simulink library "sm_trackV_lib_belt_underc_elem"  (R2026a)
settings: Solver=VariableStepAuto
undefined symbols (not defined in the file): Excv, P00, P01, P02, P03, P04, P05, P06, P07, P08, P09, P10, P11, P12, P13, P14, P15, P16, P17, P18, P19, P20, Trac, X, Y, Z
libraries: sm_lib x193, $bdroot x42
(part 1 of 5)
Description:
  | Copyright 2024-2026 The MathWorks, Inc.
settings Model: Creator=smiller  LastModifiedBy=smiller

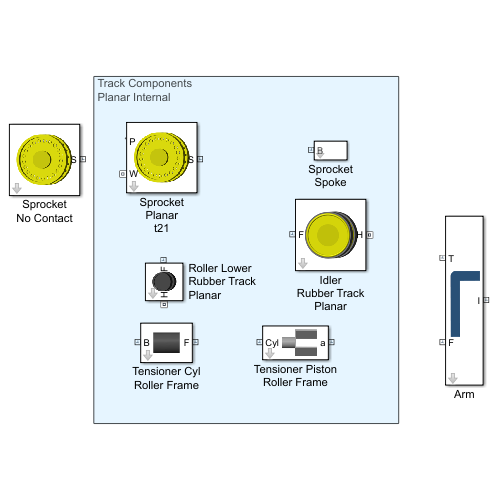
[thumbnail: Simulink's stored preview of the top-level diagram]
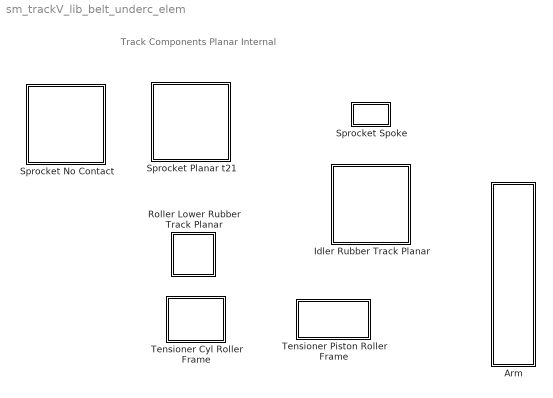
== system sm_trackV_lib_belt_underc_elem ==
  note: Track Components
      | Planar Internal
  Arm : Subsystem  mask(Idler Arm, Tracked Vehicle){arm_idlerc=Trac.IdlerArm.Pivot_to_Idler, arm_tens_x=Trac.IdlerArm.Pivot_to_TensionerX, arm_tens_y=Trac.IdlerArm.Pivot_to_TensionerY, arm_wid=Trac.IdlerArm.wid, arm_thk=Trac.IdlerArm.thk, arm_rho=Trac.IdlerArm.rho, arm_clr=Trac.IdlerArm.clr, arm_opc=Trac.IdlerArm.opc}
      mask prompts: arm_idlerc "Offset Pivot to Idler Center (m)"; arm_tens_x "Offset Pivot to Tensioner Long.  (m)"; arm_tens_y "Offset Pivot to Tensioner Vert.  (m)"; arm_wid "Idler Arm Width (m)"; arm_thk "Idler Arm Thickness (m)"; arm_rho "Idler Arm Density (kg/m^3)"; arm_clr "Idler Arm Color [R G B] (0-1)"; arm_opc "Idler Arm Opacity (0-1)"
      mask help: Models hinged idler arm for tracked vehicle. Connects idler wheel rotation axis to pivot point on lower frame and tensioner bracket.
      mask init:
      | upDown = 180*(ge(arm_tens_y,0));
      mask DialogControl Container4 Prompt: Idler Arm
      mask Display: image('sm_idler_arm_IMAGE.png')
  Idler Rubber Track Planar : Subsystem  mask(Idler, Belt Track, Planar Contact){idler_rad=Trac.IdlerF.rad, idler_len=Trac.IdlerF.len, wheel_clr=Trac.IdlerF.Wheel.clr, rim_rad=Trac.IdlerF.Rim.rad, rim_hub_rad=Trac.IdlerF.Rim.hub_rad, rim_xc=Trac.IdlerF.Rim.rim_xc, idler_rho=Trac.IdlerF.rho, idler_opc=Trac.IdlerF.opc, idler_clr=Trac.IdlerF.clr, idler_axle_rad=Trac.IdlerF.Axle.rad, idler_axle_len=Trac.IdlerF.Axle.len, idler_axle_rho=Trac.IdlerF.Axle.rho, idler_axle_opc=Trac.IdlerF.Axle.opc, idler_axle_clr=Trac.IdlerF.Axle.clr, idler_contgeo_clr=Trac.IdlerF.belt_contact.clr, idler_contgeo_opc=Trac.IdlerF.belt_contact.opc}
      mask prompts: idler_rad "Radius (m)"; idler_len "Length (m)"; wheel_clr "Wheel Color [R G B] (0-1)"; rim_rad "Radius (m)"; rim_hub_rad "Hub Radius (m)"; rim_xc "Cross Section [x y] (m)"; idler_rho "Density (kg/m^3)"; idler_opc "Opacity (0-1)"; idler_clr "Color [R G B] (0-1)"; idler_axle_rad "Radius (m)"; idler_axle_len "Length (m)"; idler_axle_rho "Density (kg/m^3)"; idler_axle_opc "Opacity (0-1)"; idler_axle_clr "Color [R G B] (0-1)"; idler_contgeo_clr "Color [R G B] (0-1)"; idler_contgeo_opc "Opacity (0-1)"
      mask help: Models idler on a rubber belt. Includes gap so lugs on belt can pass between rollers. Contact geometry assumes contact with belt is planar.
      mask init:
      | wheel_xc = [...
      |             rim_rad     -idler_len/2;
      |             idler_rad   -idler_len/2;
      |             idler_rad   idler_len/2;
      |             rim_rad     idler_len/2;
      |             ];
      mask DialogControl cont_idler_roller Prompt: Roller
      mask DialogControl cont_roller_rim Prompt: Rim
      mask DialogControl cont_idler_axle Prompt: Axle
      mask DialogControl cont_contact_geo_lower Prompt: Contact Geometry
      mask Display: image('sm_belt_idler_IMAGE.png');
  Roller Lower Rubber Track Planar : Subsystem  mask(Lower Roller, Belt Track, Planar Contact){roller_lower_rad=Trac.Roller.Lower.rad, roller_lower_len=Trac.Roller.Lower.len, roller_lower_rho=Trac.Roller.Lower.rho, roller_lower_clr=Trac.Roller.Lower.clr, roller_lower_opc=Trac.Roller.Lower.opc, roller_lower_rim_thk=Trac.Roller.Lower.rim_thk, roller_lower_rim_len=Trac.Roller.Lower.rim_len, roller_lower_axle_rad=Trac.Roller.Lower.Axle.rad, roller_lower_axle_len=Trac.Roller.Lower.Axle.len, roller_lower_axle_rho=Trac.Roller.Lower.Axle.rho, roller_lower_axle_opc=Trac.Roller.Lower.Axle.opc, roller_lower_axle_clr=Trac.Roller.Lower.Axle.clr, roller_lower_contgeo_clr=Trac.Roller.Lower.belt_contact.clr, roller_lower_contgeo_opc=Trac.Roller.Lower.belt_contact.opc}
      mask prompts: roller_lower_rad "Radius (m)"; roller_lower_len "Length (m)"; roller_lower_rho "Density (kg/m^3)"; roller_lower_clr "Color [R G B] (0-1)"; roller_lower_opc "Opacity (0-1)"; roller_lower_rim_thk "Thickness (m)"; roller_lower_rim_len "Length (m)"; roller_lower_axle_rad "Radius (m)"; roller_lower_axle_len "Length (m)"; roller_lower_axle_rho "Density (kg/m^3)"; roller_lower_axle_opc "Opacity (0-1)"; roller_lower_axle_clr "Color [R G B] (0-1)"; roller_lower_contgeo_clr "Color [R G B] (0-1)"; roller_lower_contgeo_opc "Opacity (0-1)"
      mask help: Models roller for use on rubber belt. Includes gap so lugs on belt can pass through. Contact geometry assumes contact with belt is planar.
      mask init:
      | roller_xc = [...
      |     0 -roller_lower_len/2+roller_lower_rim_len;...
      |     roller_lower_rad-roller_lower_rim_thk -roller_lower_len/2+roller_lower_rim_len;...
      |     roller_lower_rad-roller_lower_rim_thk -roller_lower_len/2;...
      |     roller_lower_rad                      -roller_lower_len/2;...
      |     roller_lower_rad                       roller_lower_len/2;...
      |     roller_lower_rad-roller_lower_rim_thk  roller_lower_len/2;...
      |     0                                      roller_lower_len/2];
      mask DialogControl cont_roller_lower Prompt: Roller
      mask DialogControl cont_rollerL_rim Prompt: Rim
      mask DialogControl cont_roller_lower_axle Prompt: Axle
      mask DialogControl cont_contact_geo_lower Prompt: Contact Geometry
      mask Display: image('sm_belt_roller_IMAGE.png');
  Sprocket No Contact : Subsystem  mask(Sprocket Wheel, Belt Track, Planar Contact){sprk_wid_roll=Trac.Sprocket.Roller.wid, sprk_rad_roll=Trac.Sprocket.Roller.rad, sprk_opc=Trac.Sprocket.Roller.opc, sprk_clr=Trac.Sprocket.Roller.clr, sprk_rad_pitch=Trac.Sprocket.Spoke.pitch_rad, sprk_spoke_rad=Trac.Sprocket.Spoke.rad, sprk_spoke_len=Trac.Sprocket.Spoke.len, sprk_spoke_num=Trac.Sprocket.nSpokes, sprk_spoke_clr=Trac.Sprocket.Spoke.clr, sprk_spoke_opc=Trac.Sprocket.Spoke.opc, rim_spoke_xc=Trac.Sprocket.Rim.spoke_xc, rim_thk=Trac.Sprocket.Rim.thk, rim_ir=Trac.Sprocket.Rim.rad_inner}
      mask prompts: sprk_wid_roll "Roller Width (m)"; sprk_rad_roll "Rolling Radius (m)"; sprk_opc "Roller Opacity (0-1)"; sprk_clr "Roller Color [R G B] (0-1)"; sprk_rad_pitch "Pitch Radius (m)"; sprk_spoke_rad "Radius (m)"; sprk_spoke_len "Length (m)"; sprk_spoke_num "Number of Spokes"; sprk_spoke_clr "Spoke Color [R G B] (0-1)"; sprk_spoke_opc "Spoke Opacity (0-1)"; rim_spoke_xc "Spoke Cross Section [x y] (m)"; rim_thk "Thickness (m)"; rim_ir "Inner Radius (m)"
      mask help: Models sprocket for belt track. Pins contact lugs on belt, rollers contact belt. Contact geometry assumes contact with belt and lugs is planar.
      mask DialogControl cont_sprkt Prompt: Sprocket
      mask DialogControl cont_sprk_roller Prompt: Roller
      mask DialogControl cont_sprk_spoke Prompt: Spoke
      mask DialogControl cont_sprk_rim Prompt: Rim
      mask Display: image('sm_belt_sprocket_IMAGE.png')
  Sprocket Planar t21 : Subsystem  mask(Sprocket Wheel, Belt Track, Planar Contact){sprk_wid_roll=Trac.Sprocket.Roller.wid, sprk_rad_roll=Trac.Sprocket.Roller.rad, sprk_opc=Trac.Sprocket.Roller.opc, sprk_clr=Trac.Sprocket.Roller.clr, sprk_rad_pitch=Trac.Sprocket.Spoke.pitch_rad, sprk_spoke_rad=Trac.Sprocket.Spoke.rad, sprk_spoke_len=Trac.Sprocket.Spoke.len, sprk_spoke_num=Trac.Sprocket.nSpokes, sprk_spoke_clr=Trac.Sprocket.Spoke.clr, sprk_spoke_opc=Trac.Sprocket.Spoke.opc, rim_spoke_xc=Trac.Sprocket.Rim.spoke_xc, rim_thk=Trac.Sprocket.Rim.thk, rim_ir=Trac.Sprocket.Rim.rad_inner, sprk_contgeo_roller_clr=Trac.Sprocket.roller_contact.clr, sprk_contgeo_roller_opc=Trac.Sprocket.roller_contact.opc, sprk_contgeo_spoke_clr=Trac.Sprocket.spoke_contact.clr, sprk_contgeo_spoke_opc=Trac.Sprocket.spoke_contact.opc}
      mask prompts: sprk_wid_roll "Roller Width (m)"; sprk_rad_roll "Rolling Radius (m)"; sprk_opc "Roller Opacity (0-1)"; sprk_clr "Roller Color [R G B] (0-1)"; sprk_rad_pitch "Pitch Radius (m)"; sprk_spoke_rad "Radius (m)"; sprk_spoke_len "Length (m)"; sprk_spoke_num "Number of Spokes"; sprk_spoke_clr "Spoke Color [R G B] (0-1)"; sprk_spoke_opc "Spoke Opacity (0-1)"; rim_spoke_xc "Spoke Cross Section [x y] (m)"; rim_thk "Thickness (m)"; rim_ir "Inner Radius (m)"; sprk_contgeo_roller_clr "Roller Color [R G B] (0-1)"; sprk_contgeo_roller_opc "Roller Opacity (0-1)"; sprk_contgeo_spoke_clr "Spoke Color [R G B] (0-1)"; sprk_contgeo_spoke_opc "Spoke Opacity (0-1)"
      mask help: Models sprocket for belt track. Pins contact lugs on belt, rollers contact belt. Contact geometry assumes contact with belt and lugs is planar.
      mask DialogControl cont_sprkt Prompt: Sprocket
      mask DialogControl cont_sprk_roller Prompt: Roller
      mask DialogControl cont_sprk_spoke Prompt: Spoke
      mask DialogControl cont_sprk_rim Prompt: Rim
      mask DialogControl cont_sprk_contgeo Prompt: Contact Geometry
      mask Display: image('sm_belt_sprocket_IMAGE.png')
  Sprocket Spoke : Subsystem  mask(Spoke on Sprocket Wheel){spoke_xc=Trac.Sprocket.xc_spoke, spoke_thk=Trac.Sprocket.spoke_thk, spoke_clr=Trac.Sprocket.Roller.clr, spoke_opc=Trac.Sprocket.Roller.opc, sprk_pin_len=Trac.Sprocket.Spoke.len}
      mask prompts: spoke_xc "Spoke Cross-Section [x y] (m)"; spoke_thk "Spoke Thickness (m)"; spoke_clr "Spoke Color [R G B] (0-1)"; spoke_opc "Spoke Color (0-1)"; sprk_pin_len "Sprocket Pin Length (m)"
      mask help: Models geometry of spoke in sprocket wheel. Spoke has pin at midpoint outer edge.
      mask init:
      | spoke_offset = (sprk_pin_len+spoke_thk)/2;
      mask TypeOptions spoke_xc: Spoke nz/ExtrusionCrossSection | Spoke pz/ExtrusionCrossSection
      mask TypeOptions spoke_thk: Spoke nz/ExtrusionLength | Spoke pz/ExtrusionLength
      mask TypeOptions spoke_clr: Spoke nz/GraphicDiffuseColor | Spoke pz/GraphicDiffuseColor
      mask TypeOptions spoke_opc: Spoke nz/GraphicOpacity | Spoke pz/GraphicOpacity
  Tensioner Cyl Roller Frame : Subsystem  mask(Tensioner Cylinder){cyl_rad=Excv.Idler.Tensioner.cyl.rad, cyl_len=Excv.Idler.Tensioner.cyl.len, cyl_rho=Excv.Idler.Tensioner.cyl.rho, cyl_clr=Excv.Idler.Tensioner.cyl.clr, cyl_opc=Excv.Idler.Tensioner.cyl.opc}
      mask prompts: cyl_rad "Radius (m)"; cyl_len "Length (m)"; cyl_rho "Density (kg/m^3)"; cyl_clr "Color [R G B] (0-1)"; cyl_opc "Opacity (0-1)"
      mask help: Models tensioner cylinder in undercarriage.
      mask DialogControl cont_cyl Prompt: Cylinder
      mask Display: image('sm_chain_tensioner_cyl_IMAGE.png');
  Tensioner Piston Roller Frame : Subsystem  mask(Tensioner Piston and Bracket){pist_rad=Excv.Idler.Tensioner.piston.rad, pist_len=Excv.Idler.Tensioner.piston.len, pist_rho=Excv.Idler.Tensioner.piston.rho, pist_clr=Excv.Idler.Tensioner.piston.clr, pist_opc=Excv.Idler.Tensioner.piston.opc, br_height=Excv.Idler.Tensioner.bracket.height, br_length=Excv.Idler.Tensioner.bracket.len, br_width=Excv.Idler.Tensioner.bracket.wid, br_rho=Excv.Idler.Tensioner.bracket.rho, br_thk=Excv.Idler.Tensioner.bracket.thk, br_clr=Excv.Idler.Tensioner.bracket.clr, br_opc=Excv.Idler.Tensioner.bracket.opc}
      mask prompts: pist_rad "Radius (m)"; pist_len "Length (m)"; pist_rho "Density (kg/m^3)"; pist_clr "Color [R G B] (0-1)"; pist_opc "Opacity (0.1)"; br_height "Height (m)"; br_length "Length (m)"; br_width "Width (m)"; br_rho "Density (kg/m^3)"; br_thk "Thickness (m)"; br_clr "Color [R G B] (0-1)"; br_opc "Opacity (0.1)"
      mask help: Models tensioner piston and bracket in undercarriage.
      mask DialogControl cont_piston Prompt: Piston
      mask DialogControl cont_bracket Prompt: Bracket
      mask Display: image('sm_chain_tensioner_piston_IMAGE.png');

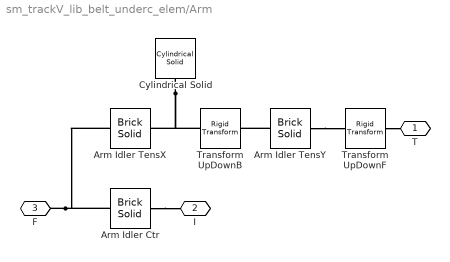
== system sm_trackV_lib_belt_underc_elem/Arm ==
  Arm Idler Ctr : sm_lib/Body Elements/Brick Solid  BrickDimensions=[arm_idlerc arm_wid arm_thk]  BrickDimensionsUnits=m  ExportEntireGeometry=off  InertiaType=CalculateFromGeometry  BasedOnType=Density  Density=arm_rho  DensityUnits=kg/m^3  Mass=1  MassUnits=kg  CenterOfMass=[0 0 0]  CenterOfMassUnits=m  MomentsOfInertia=[1 1 1]  MomentsOfInertiaUnits=kg*m^2  ProductsOfInertia=[0 0 0]  ProductsOfInertiaUnits=kg*m^2  GraphicType=FromGeometry  MarkerShape=Sphere  MarkerSize=10  GraphicVisPropType=SimpleVisualProperties  GraphicDiffuseColor=arm_clr  GraphicOpacity=arm_opc  GraphicSpecularColor=[0.5 0.5 0.5 1.0]  GraphicAmbientColor=[0.15 0.15 0.15 1.0]  GraphicEmissiveColor=[0.0 0.0 0.0 1.0]  GraphicShininess=75  DoExposeReferenceFrame=off  SerializedFrames=<Frames><Frame><Id>Frame1</Id><Value><Name>B</Name><Origin><Source>GeometricFeature</Source><FeatureName>-x surface</FeatureName></Origin><PrimaryAxis><DefinedDirection>+Z</DefinedDirection><Source>ReferenceFrame</Source><SourceDirection>+Z</SourceDirection><FeatureName></FeatureName></PrimaryAxis><SecondaryAxis><DefinedDirection>+X</DefinedDirection><Source>ReferenceFrame</Source><SourceDirection>+X</SourceDirection><FeatureName></FeatureName></SecondaryAxis></Value></Frame><Frame><Id>Frame2</Id><Value><Name>F</Name><Origin><Source>GeometricFeature</Source><FeatureName>+x surface</FeatureName></Origin><PrimaryAxis><DefinedDirection>+Z</DefinedDirection><Source>ReferenceFrame</Source><SourceDirection>+Z</SourceDirection><FeatureName></FeatureName></PrimaryAxis><SecondaryAxis><DefinedDirection>+X</DefinedDirection><Source>ReferenceFrame</Source><SourceDirection>+X</SourceDirection><FeatureName></FeatureName></SecondaryAxis></Value></Frame></Frames>
  Arm Idler TensX : sm_lib/Body Elements/Brick Solid  BrickDimensions=[arm_tens_x arm_wid arm_thk]  BrickDimensionsUnits=m  ExportEntireGeometry=off  InertiaType=CalculateFromGeometry  BasedOnType=Density  Density=arm_rho  DensityUnits=kg/m^3  Mass=1  MassUnits=kg  CenterOfMass=[0 0 0]  CenterOfMassUnits=m  MomentsOfInertia=[1 1 1]  MomentsOfInertiaUnits=kg*m^2  ProductsOfInertia=[0 0 0]  ProductsOfInertiaUnits=kg*m^2  GraphicType=FromGeometry  MarkerShape=Sphere  MarkerSize=10  GraphicVisPropType=SimpleVisualProperties  GraphicDiffuseColor=arm_clr  GraphicOpacity=arm_opc  GraphicSpecularColor=[0.5 0.5 0.5 1.0]  GraphicAmbientColor=[0.15 0.15 0.15 1.0]  GraphicEmissiveColor=[0.0 0.0 0.0 1.0]  GraphicShininess=75  DoExposeReferenceFrame=off  SerializedFrames=<Frames><Frame><Id>Frame1</Id><Value><Name>B</Name><Origin><Source>GeometricFeature</Source><FeatureName>-x surface</FeatureName></Origin><PrimaryAxis><DefinedDirection>+Z</DefinedDirection><Source>ReferenceFrame</Source><SourceDirection>+Z</SourceDirection><FeatureName></FeatureName></PrimaryAxis><SecondaryAxis><DefinedDirection>+X</DefinedDirection><Source>ReferenceFrame</Source><SourceDirection>+X</SourceDirection><FeatureName></FeatureName></SecondaryAxis></Value></Frame><Frame><Id>Frame2</Id><Value><Name>F</Name><Origin><Source>GeometricFeature</Source><FeatureName>+x surface</FeatureName></Origin><PrimaryAxis><DefinedDirection>+Z</DefinedDirection><Source>ReferenceFrame</Source><SourceDirection>+Z</SourceDirection><FeatureName></FeatureName></PrimaryAxis><SecondaryAxis><DefinedDirection>+X</DefinedDirection><Source>ReferenceFrame</Source><SourceDirection>+X</SourceDirection><FeatureName></FeatureName></SecondaryAxis></Value></Frame></Frames>
  Arm Idler TensY : sm_lib/Body Elements/Brick Solid  BrickDimensions=[arm_wid abs(arm_tens_y) arm_thk]  BrickDimensionsUnits=m  ExportEntireGeometry=off  InertiaType=CalculateFromGeometry  BasedOnType=Density  Density=arm_rho  DensityUnits=kg/m^3  Mass=1  MassUnits=kg  CenterOfMass=[0 0 0]  CenterOfMassUnits=m  MomentsOfInertia=[1 1 1]  MomentsOfInertiaUnits=kg*m^2  ProductsOfInertia=[0 0 0]  ProductsOfInertiaUnits=kg*m^2  GraphicType=FromGeometry  MarkerShape=Sphere  MarkerSize=10  GraphicVisPropType=SimpleVisualProperties  GraphicDiffuseColor=arm_clr  GraphicOpacity=arm_opc  GraphicSpecularColor=[0.5 0.5 0.5 1.0]  GraphicAmbientColor=[0.15 0.15 0.15 1.0]  GraphicEmissiveColor=[0.0 0.0 0.0 1.0]  GraphicShininess=75  DoExposeReferenceFrame=off  SerializedFrames=<Frames><Frame><Id>Frame1</Id><Value><Name>B</Name><Origin><Source>GeometricFeature</Source><FeatureName>+y surface</FeatureName></Origin><PrimaryAxis><DefinedDirection>+Z</DefinedDirection><Source>ReferenceFrame</Source><SourceDirection>+Z</SourceDirection><FeatureName></FeatureName></PrimaryAxis><SecondaryAxis><DefinedDirection>+X</DefinedDirection><Source>ReferenceFrame</Source><SourceDirection>+X</SourceDirection><FeatureName></FeatureName></SecondaryAxis></Value></Frame><Frame><Id>Frame2</Id><Value><Name>F</Name><Origin><Source>GeometricFeature</Source><FeatureName>-y surface</FeatureName></Origin><PrimaryAxis><DefinedDirection>+Z</DefinedDirection><Source>ReferenceFrame</Source><SourceDirection>+Z</SourceDirection><FeatureName></FeatureName></PrimaryAxis><SecondaryAxis><DefinedDirection>+X</DefinedDirection><Source>ReferenceFrame</Source><SourceDirection>+X</SourceDirection><FeatureName></FeatureName></SecondaryAxis></Value></Frame></Frames>
  Cylindrical Solid : sm_lib/Body Elements/Cylindrical Solid  CylinderRadius=arm_wid/2  CylinderRadiusUnits=m  CylinderLength=arm_thk  CylinderLengthUnits=m  ExportEntireGeometry=off  InertiaType=CalculateFromGeometry  BasedOnType=Density  Density=arm_rho  DensityUnits=kg/m^3  Mass=1  MassUnits=kg  CenterOfMass=[0 0 0]  CenterOfMassUnits=m  MomentsOfInertia=[1 1 1]  MomentsOfInertiaUnits=kg*m^2  ProductsOfInertia=[0 0 0]  ProductsOfInertiaUnits=kg*m^2  GraphicType=FromGeometry  MarkerShape=Sphere  MarkerSize=10  GraphicVisPropType=SimpleVisualProperties  GraphicDiffuseColor=arm_clr  GraphicOpacity=arm_opc  GraphicSpecularColor=[0.5 0.5 0.5 1.0]  GraphicAmbientColor=[0.15 0.15 0.15 1.0]  GraphicEmissiveColor=[0.0 0.0 0.0 1.0]  GraphicShininess=75  DoExposeReferenceFrame=on  SerializedFrames=<Frames/>
  Transform UpDownB : sm_lib/Frames and Transforms/Rigid Transform  RotationMethod=StandardAxis  FollAlignAxisA=+X  BaseAlignAxisA=+Y  FollAlignAxisB=+Y  BaseAlignAxisB=+Z  RotationStandardAxis=+X  RotationAngle=upDown  RotationAngleUnits=deg  RotationArbitraryAxis=[0 0 1]  RotationSequenceAxes=FollowerAxes  RotationSequence=XYX  RotationSequenceAngles=[0 0 0]  RotationSequenceAnglesUnits=deg  RotationMatrix=[1 0 0; 0 1 0; 0 0 1]  Quaternion=[1 0 0 0]  TranslationMethod=None  TranslationCartesianOffset=[0 0 0]  TranslationCartesianOffsetUnits=m  TranslationStandardAxis=+Z  TranslationStandardOffset=0  TranslationStandardOffsetUnits=m  TranslationROffset=0  TranslationROffsetUnits=m  TranslationThetaOffset=0  TranslationThetaOffsetUnits=deg  TranslationZOffset=0  TranslationZOffsetUnits=m
  Transform UpDownF : sm_lib/Frames and Transforms/Rigid Transform  RotationMethod=StandardAxis  FollAlignAxisA=+X  BaseAlignAxisA=+Y  FollAlignAxisB=+Y  BaseAlignAxisB=+Z  RotationStandardAxis=+X  RotationAngle=upDown  RotationAngleUnits=deg  RotationArbitraryAxis=[0 0 1]  RotationSequenceAxes=FollowerAxes  RotationSequence=XYX  RotationSequenceAngles=[0 0 0]  RotationSequenceAnglesUnits=deg  RotationMatrix=[1 0 0; 0 1 0; 0 0 1]  Quaternion=[1 0 0 0]  TranslationMethod=None  TranslationCartesianOffset=[0 0 0]  TranslationCartesianOffsetUnits=m  TranslationStandardAxis=+Z  TranslationStandardOffset=0  TranslationStandardOffsetUnits=m  TranslationROffset=0  TranslationROffsetUnits=m  TranslationThetaOffset=0  TranslationThetaOffsetUnits=deg  TranslationZOffset=0  TranslationZOffsetUnits=m
  T : PMIOPort  Side=Left
  I : PMIOPort  Port=2  Side=Right
  F : PMIOPort  Port=3  Side=Left
  connections:
  Cylindrical Solid/RConn1 -- Arm Idler TensX/RConn1 -- Transform UpDownB/LConn1
  Arm Idler Ctr/RConn1 -- I/RConn1
  F/RConn1 -- Arm Idler TensX/LConn1 -- Arm Idler Ctr/LConn1
  Arm Idler TensY/RConn1 -- Transform UpDownF/RConn1
  Transform UpDownF/LConn1 -- T/RConn1
  Arm Idler TensY/LConn1 -- Transform UpDownB/RConn1

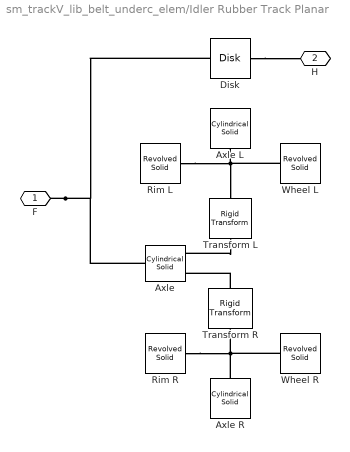
== system sm_trackV_lib_belt_underc_elem/Idler Rubber Track Planar ==
  Axle : sm_lib/Body Elements/Cylindrical Solid  CylinderRadius=idler_axle_rad  CylinderRadiusUnits=m  CylinderLength=idler_axle_len  CylinderLengthUnits=m  ExportEntireGeometry=off  InertiaType=CalculateFromGeometry  BasedOnType=Density  Density=idler_axle_rho  DensityUnits=kg/m^3  Mass=1  MassUnits=kg  CenterOfMass=[0 0 0]  CenterOfMassUnits=m  MomentsOfInertia=[1 1 1]  MomentsOfInertiaUnits=kg*m^2  ProductsOfInertia=[0 0 0]  ProductsOfInertiaUnits=kg*m^2  GraphicType=FromGeometry  MarkerShape=Sphere  MarkerSize=10  GraphicVisPropType=SimpleVisualProperties  GraphicDiffuseColor=idler_axle_clr  GraphicOpacity=idler_axle_opc  GraphicSpecularColor=[0.5 0.5 0.5 1.0]  GraphicAmbientColor=[0.15 0.15 0.15 1.0]  GraphicEmissiveColor=[0.0 0.0 0.0 1.0]  GraphicShininess=75  DoExposeReferenceFrame=on  SerializedFrames=<Frames><Frame><Id>Frame1</Id><Value><Name>F</Name><Origin><Source>GeometricFeature</Source><FeatureName>top surface</FeatureName></Origin><PrimaryAxis><DefinedDirection>+Z</DefinedDirection><Source>ReferenceFrame</Source><SourceDirection>+Z</SourceDirection><FeatureName></FeatureName></PrimaryAxis><SecondaryAxis><DefinedDirection>+X</DefinedDirection><Source>ReferenceFrame</Source><SourceDirection>+X</SourceDirection><FeatureName></FeatureName></SecondaryAxis></Value></Frame><Frame><Id>Frame2</Id><Value><Name>B</Name><Origin><Source>GeometricFeature</Source><FeatureName>bottom surface</FeatureName></Origin><PrimaryAxis><DefinedDirection>+Z</DefinedDirection><Source>ReferenceFrame</Source><SourceDirection>+Z</SourceDirection><FeatureName></FeatureName></PrimaryAxis><SecondaryAxis><DefinedDirection>+X</DefinedDirection><Source>ReferenceFrame</Source><SourceDirection>+X</SourceDirection><FeatureName></FeatureName></SecondaryAxis></Value></Frame></Frames>
  Axle L : sm_lib/Body Elements/Cylindrical Solid  CylinderRadius=rim_hub_rad  CylinderRadiusUnits=m  CylinderLength=max(rim_xc(:,2))*2  CylinderLengthUnits=m  ExportEntireGeometry=off  InertiaType=CalculateFromGeometry  BasedOnType=Density  Density=idler_rho  DensityUnits=kg/m^3  Mass=1  MassUnits=kg  CenterOfMass=[0 0 0]  CenterOfMassUnits=m  MomentsOfInertia=[1 1 1]  MomentsOfInertiaUnits=kg*m^2  ProductsOfInertia=[0 0 0]  ProductsOfInertiaUnits=kg*m^2  GraphicType=FromGeometry  MarkerShape=Sphere  MarkerSize=10  GraphicVisPropType=SimpleVisualProperties  GraphicDiffuseColor=idler_clr*0.9  GraphicOpacity=idler_opc  GraphicSpecularColor=[0.5 0.5 0.5 1.0]  GraphicAmbientColor=[0.15 0.15 0.15 1.0]  GraphicEmissiveColor=[0.0 0.0 0.0 1.0]  GraphicShininess=75  DoExposeReferenceFrame=on  SerializedFrames=<Frames/>
  Axle R : sm_lib/Body Elements/Cylindrical Solid  CylinderRadius=rim_hub_rad  CylinderRadiusUnits=m  CylinderLength=max(rim_xc(:,2))*2  CylinderLengthUnits=m  ExportEntireGeometry=off  InertiaType=CalculateFromGeometry  BasedOnType=Density  Density=idler_rho  DensityUnits=kg/m^3  Mass=1  MassUnits=kg  CenterOfMass=[0 0 0]  CenterOfMassUnits=m  MomentsOfInertia=[1 1 1]  MomentsOfInertiaUnits=kg*m^2  ProductsOfInertia=[0 0 0]  ProductsOfInertiaUnits=kg*m^2  GraphicType=FromGeometry  MarkerShape=Sphere  MarkerSize=10  GraphicVisPropType=SimpleVisualProperties  GraphicDiffuseColor=idler_clr*0.9  GraphicOpacity=idler_opc  GraphicSpecularColor=[0.5 0.5 0.5 1.0]  GraphicAmbientColor=[0.15 0.15 0.15 1.0]  GraphicEmissiveColor=[0.0 0.0 0.0 1.0]  GraphicShininess=75  DoExposeReferenceFrame=on  SerializedFrames=<Frames/>
  Disk : sm_lib/Curves and Surfaces/Disk  Radius=idler_rad  RadiusUnits=m  GraphicType=FromGeometry  GraphicVisPropType=SimpleVisualProperties  GraphicDiffuseColor=idler_contgeo_clr  GraphicOpacity=idler_contgeo_opc  GraphicSpecularColor=[0.5 0.5 0.5 1.0]  GraphicAmbientColor=[0.15 0.15 0.15 1.0]  GraphicEmissiveColor=[0.0 0.0 0.0 1.0]  GraphicShininess=75
  Rim L : sm_lib/Body Elements/Revolved Solid  RevolutionCrossSection=rim_xc  RevolutionCrossSectionUnits=m  RevolutionExtent=Full  RevolutionAngle=180  RevolutionAngleUnits=deg  ExportConvexHullGeometry=off  InertiaType=CalculateFromGeometry  BasedOnType=Density  Density=idler_rho  DensityUnits=kg/m^3  Mass=1  MassUnits=kg  CenterOfMass=[0 0 0]  CenterOfMassUnits=m  MomentsOfInertia=[1 1 1]  MomentsOfInertiaUnits=kg*m^2  ProductsOfInertia=[0 0 0]  ProductsOfInertiaUnits=kg*m^2  GraphicType=FromGeometry  MarkerShape=Sphere  MarkerSize=10  GraphicVisPropType=SimpleVisualProperties  GraphicDiffuseColor=idler_clr  GraphicOpacity=idler_opc  GraphicSpecularColor=[0.5 0.5 0.5 1.0]  GraphicAmbientColor=[0.15 0.15 0.15 1.0]  GraphicEmissiveColor=[0.0 0.0 0.0 1.0]  GraphicShininess=75  DoExposeReferenceFrame=on  SerializedFrames=<Frames/>
  Rim R : sm_lib/Body Elements/Revolved Solid  RevolutionCrossSection=rim_xc  RevolutionCrossSectionUnits=m  RevolutionExtent=Full  RevolutionAngle=180  RevolutionAngleUnits=deg  ExportConvexHullGeometry=off  InertiaType=CalculateFromGeometry  BasedOnType=Density  Density=idler_rho  DensityUnits=kg/m^3  Mass=1  MassUnits=kg  CenterOfMass=[0 0 0]  CenterOfMassUnits=m  MomentsOfInertia=[1 1 1]  MomentsOfInertiaUnits=kg*m^2  ProductsOfInertia=[0 0 0]  ProductsOfInertiaUnits=kg*m^2  GraphicType=FromGeometry  MarkerShape=Sphere  MarkerSize=10  GraphicVisPropType=SimpleVisualProperties  GraphicDiffuseColor=idler_clr  GraphicOpacity=idler_opc  GraphicSpecularColor=[0.5 0.5 0.5 1.0]  GraphicAmbientColor=[0.15 0.15 0.15 1.0]  GraphicEmissiveColor=[0.0 0.0 0.0 1.0]  GraphicShininess=75  DoExposeReferenceFrame=on  SerializedFrames=<Frames/>
  Transform L : sm_lib/Frames and Transforms/Rigid Transform  RotationMethod=None  FollAlignAxisA=+X  BaseAlignAxisA=+Y  FollAlignAxisB=+Y  BaseAlignAxisB=+Z  RotationStandardAxis=+Z  RotationAngle=0.0  RotationAngleUnits=deg  RotationArbitraryAxis=[0 0 1]  RotationSequenceAxes=FollowerAxes  RotationSequence=XYX  RotationSequenceAngles=[0 0 0]  RotationSequenceAnglesUnits=deg  RotationMatrix=[1 0 0; 0 1 0; 0 0 1]  Quaternion=[1 0 0 0]  TranslationMethod=StandardAxis  TranslationCartesianOffset=[0 0 0]  TranslationCartesianOffsetUnits=m  TranslationStandardAxis=+Z  TranslationStandardOffset=idler_len/2  TranslationStandardOffsetUnits=m  TranslationROffset=0  TranslationROffsetUnits=m  TranslationThetaOffset=0  TranslationThetaOffsetUnits=deg  TranslationZOffset=0  TranslationZOffsetUnits=m
  Transform R : sm_lib/Frames and Transforms/Rigid Transform  RotationMethod=None  FollAlignAxisA=+X  BaseAlignAxisA=+Y  FollAlignAxisB=+Y  BaseAlignAxisB=+Z  RotationStandardAxis=+Z  RotationAngle=0.0  RotationAngleUnits=deg  RotationArbitraryAxis=[0 0 1]  RotationSequenceAxes=FollowerAxes  RotationSequence=XYX  RotationSequenceAngles=[0 0 0]  RotationSequenceAnglesUnits=deg  RotationMatrix=[1 0 0; 0 1 0; 0 0 1]  Quaternion=[1 0 0 0]  TranslationMethod=StandardAxis  TranslationCartesianOffset=[0 0 0]  TranslationCartesianOffsetUnits=m  TranslationStandardAxis=-Z  TranslationStandardOffset=idler_len/2  TranslationStandardOffsetUnits=m  TranslationROffset=0  TranslationROffsetUnits=m  TranslationThetaOffset=0  TranslationThetaOffsetUnits=deg  TranslationZOffset=0  TranslationZOffsetUnits=m
  Wheel L : sm_lib/Body Elements/Revolved Solid  RevolutionCrossSection=wheel_xc  RevolutionCrossSectionUnits=m  RevolutionExtent=Full  RevolutionAngle=180  RevolutionAngleUnits=deg  ExportConvexHullGeometry=off  InertiaType=CalculateFromGeometry  BasedOnType=Density  Density=idler_rho  DensityUnits=kg/m^3  Mass=1  MassUnits=kg  CenterOfMass=[0 0 0]  CenterOfMassUnits=m  MomentsOfInertia=[1 1 1]  MomentsOfInertiaUnits=kg*m^2  ProductsOfInertia=[0 0 0]  ProductsOfInertiaUnits=kg*m^2  GraphicType=FromGeometry  MarkerShape=Sphere  MarkerSize=10  GraphicVisPropType=SimpleVisualProperties  GraphicDiffuseColor=wheel_clr  GraphicOpacity=idler_opc  GraphicSpecularColor=[0.5 0.5 0.5 1.0]  GraphicAmbientColor=[0.15 0.15 0.15 1.0]  GraphicEmissiveColor=[0.0 0.0 0.0 1.0]  GraphicShininess=75  DoExposeReferenceFrame=on  SerializedFrames=<Frames/>
  Wheel R : sm_lib/Body Elements/Revolved Solid  RevolutionCrossSection=wheel_xc  RevolutionCrossSectionUnits=m  RevolutionExtent=Full  RevolutionAngle=180  RevolutionAngleUnits=deg  ExportConvexHullGeometry=off  InertiaType=CalculateFromGeometry  BasedOnType=Density  Density=idler_rho  DensityUnits=kg/m^3  Mass=1  MassUnits=kg  CenterOfMass=[0 0 0]  CenterOfMassUnits=m  MomentsOfInertia=[1 1 1]  MomentsOfInertiaUnits=kg*m^2  ProductsOfInertia=[0 0 0]  ProductsOfInertiaUnits=kg*m^2  GraphicType=FromGeometry  MarkerShape=Sphere  MarkerSize=10  GraphicVisPropType=SimpleVisualProperties  GraphicDiffuseColor=wheel_clr  GraphicOpacity=idler_opc  GraphicSpecularColor=[0.5 0.5 0.5 1.0]  GraphicAmbientColor=[0.15 0.15 0.15 1.0]  GraphicEmissiveColor=[0.0 0.0 0.0 1.0]  GraphicShininess=75  DoExposeReferenceFrame=on  SerializedFrames=<Frames/>
  F : PMIOPort  Side=Left
  H : PMIOPort  Port=2  Side=Right
  connections:
  Transform L/LConn1 -- Axle/LConn1
  Transform R/LConn1 -- Axle/LConn2
  F/RConn1 -- Disk/LConn1 -- Axle/RConn1
  Disk/RConn1 -- H/RConn1
  Rim L/RConn1 -- Transform L/RConn1 -- Axle L/RConn1 -- Wheel L/RConn1
  Wheel R/RConn1 -- Axle R/RConn1 -- Transform R/RConn1 -- Rim R/RConn1

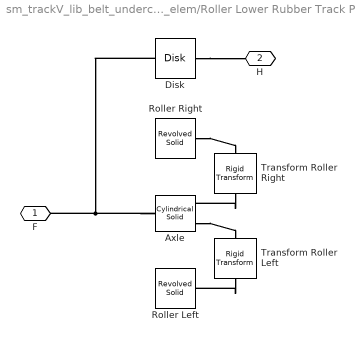
== system sm_trackV_lib_belt_underc_elem/Roller Lower Rubber Track Planar ==
  Axle : sm_lib/Body Elements/Cylindrical Solid  CylinderRadius=roller_lower_axle_rad  CylinderRadiusUnits=m  CylinderLength=roller_lower_axle_len  CylinderLengthUnits=m  ExportEntireGeometry=off  InertiaType=CalculateFromGeometry  BasedOnType=Density  Density=roller_lower_axle_rho  DensityUnits=kg/m^3  Mass=1  MassUnits=kg  CenterOfMass=[0 0 0]  CenterOfMassUnits=m  MomentsOfInertia=[1 1 1]  MomentsOfInertiaUnits=kg*m^2  ProductsOfInertia=[0 0 0]  ProductsOfInertiaUnits=kg*m^2  GraphicType=FromGeometry  MarkerShape=Sphere  MarkerSize=10  GraphicVisPropType=SimpleVisualProperties  GraphicDiffuseColor=roller_lower_axle_clr  GraphicOpacity=roller_lower_axle_opc  GraphicSpecularColor=[0.5 0.5 0.5 1.0]  GraphicAmbientColor=[0.15 0.15 0.15 1.0]  GraphicEmissiveColor=[0.0 0.0 0.0 1.0]  GraphicShininess=75  DoExposeReferenceFrame=on  SerializedFrames=<Frames><Frame><Id>Frame1</Id><Value><Name>F</Name><Origin><Source>GeometricFeature</Source><FeatureName>top surface</FeatureName></Origin><PrimaryAxis><DefinedDirection>+Z</DefinedDirection><Source>ReferenceFrame</Source><SourceDirection>+Z</SourceDirection><FeatureName></FeatureName></PrimaryAxis><SecondaryAxis><DefinedDirection>+X</DefinedDirection><Source>ReferenceFrame</Source><SourceDirection>+X</SourceDirection><FeatureName></FeatureName></SecondaryAxis></Value></Frame><Frame><Id>Frame2</Id><Value><Name>B</Name><Origin><Source>GeometricFeature</Source><FeatureName>bottom surface</FeatureName></Origin><PrimaryAxis><DefinedDirection>+Z</DefinedDirection><Source>ReferenceFrame</Source><SourceDirection>+Z</SourceDirection><FeatureName></FeatureName></PrimaryAxis><SecondaryAxis><DefinedDirection>+X</DefinedDirection><Source>ReferenceFrame</Source><SourceDirection>+X</SourceDirection><FeatureName></FeatureName></SecondaryAxis></Value></Frame></Frames>
  Disk : sm_lib/Curves and Surfaces/Disk  Radius=roller_lower_rad  RadiusUnits=m  GraphicType=FromGeometry  GraphicVisPropType=SimpleVisualProperties  GraphicDiffuseColor=roller_lower_contgeo_clr  GraphicOpacity=roller_lower_contgeo_opc  GraphicSpecularColor=[0.5 0.5 0.5 1.0]  GraphicAmbientColor=[0.15 0.15 0.15 1.0]  GraphicEmissiveColor=[0.0 0.0 0.0 1.0]  GraphicShininess=75
  Roller Left : sm_lib/Body Elements/Revolved Solid  RevolutionCrossSection=roller_xc  RevolutionCrossSectionUnits=m  RevolutionExtent=Full  RevolutionAngle=180  RevolutionAngleUnits=deg  ExportConvexHullGeometry=off  InertiaType=CalculateFromGeometry  BasedOnType=Density  Density=roller_lower_rho  DensityUnits=kg/m^3  Mass=1  MassUnits=kg  CenterOfMass=[0 0 0]  CenterOfMassUnits=m  MomentsOfInertia=[1 1 1]  MomentsOfInertiaUnits=kg*m^2  ProductsOfInertia=[0 0 0]  ProductsOfInertiaUnits=kg*m^2  GraphicType=FromGeometry  MarkerShape=Sphere  MarkerSize=10  GraphicVisPropType=SimpleVisualProperties  GraphicDiffuseColor=roller_lower_clr  GraphicOpacity=roller_lower_opc  GraphicSpecularColor=[0.5 0.5 0.5 1.0]  GraphicAmbientColor=[0.15 0.15 0.15 1.0]  GraphicEmissiveColor=[0.0 0.0 0.0 1.0]  GraphicShininess=75  DoExposeReferenceFrame=on  SerializedFrames=<Frames/>
  Roller Right : sm_lib/Body Elements/Revolved Solid  RevolutionCrossSection=roller_xc  RevolutionCrossSectionUnits=m  RevolutionExtent=Full  RevolutionAngle=180  RevolutionAngleUnits=deg  ExportConvexHullGeometry=off  InertiaType=CalculateFromGeometry  BasedOnType=Density  Density=roller_lower_rho  DensityUnits=kg/m^3  Mass=1  MassUnits=kg  CenterOfMass=[0 0 0]  CenterOfMassUnits=m  MomentsOfInertia=[1 1 1]  MomentsOfInertiaUnits=kg*m^2  ProductsOfInertia=[0 0 0]  ProductsOfInertiaUnits=kg*m^2  GraphicType=FromGeometry  MarkerShape=Sphere  MarkerSize=10  GraphicVisPropType=SimpleVisualProperties  GraphicDiffuseColor=roller_lower_clr  GraphicOpacity=roller_lower_opc  GraphicSpecularColor=[0.5 0.5 0.5 1.0]  GraphicAmbientColor=[0.15 0.15 0.15 1.0]  GraphicEmissiveColor=[0.0 0.0 0.0 1.0]  GraphicShininess=75  DoExposeReferenceFrame=on  SerializedFrames=<Frames/>
  Transform Roller Left : sm_lib/Frames and Transforms/Rigid Transform  RotationMethod=None  FollAlignAxisA=+X  BaseAlignAxisA=+Y  FollAlignAxisB=+Y  BaseAlignAxisB=+Z  RotationStandardAxis=+Z  RotationAngle=0.0  RotationAngleUnits=deg  RotationArbitraryAxis=[0 0 1]  RotationSequenceAxes=FollowerAxes  RotationSequence=XYX  RotationSequenceAngles=[0 0 0]  RotationSequenceAnglesUnits=deg  RotationMatrix=[1 0 0; 0 1 0; 0 0 1]  Quaternion=[1 0 0 0]  TranslationMethod=StandardAxis  TranslationCartesianOffset=[0 0 0]  TranslationCartesianOffsetUnits=m  TranslationStandardAxis=+Z  TranslationStandardOffset=roller_lower_len/2  TranslationStandardOffsetUnits=m  TranslationROffset=0  TranslationROffsetUnits=m  TranslationThetaOffset=0  TranslationThetaOffsetUnits=deg  TranslationZOffset=0  TranslationZOffsetUnits=m
  Transform Roller Right : sm_lib/Frames and Transforms/Rigid Transform  RotationMethod=StandardAxis  FollAlignAxisA=+X  BaseAlignAxisA=+Y  FollAlignAxisB=+Y  BaseAlignAxisB=+Z  RotationStandardAxis=+X  RotationAngle=180  RotationAngleUnits=deg  RotationArbitraryAxis=[0 0 1]  RotationSequenceAxes=FollowerAxes  RotationSequence=XYX  RotationSequenceAngles=[0 0 0]  RotationSequenceAnglesUnits=deg  RotationMatrix=[1 0 0; 0 1 0; 0 0 1]  Quaternion=[1 0 0 0]  TranslationMethod=StandardAxis  TranslationCartesianOffset=[0 0 0]  TranslationCartesianOffsetUnits=m  TranslationStandardAxis=+Z  TranslationStandardOffset=roller_lower_len/2  TranslationStandardOffsetUnits=m  TranslationROffset=0  TranslationROffsetUnits=m  TranslationThetaOffset=0  TranslationThetaOffsetUnits=deg  TranslationZOffset=0  TranslationZOffsetUnits=m
  F : PMIOPort  Side=Left
  H : PMIOPort  Port=2  Side=Right
  connections:
  Disk/RConn1 -- H/RConn1
  Axle/RConn1 -- Disk/LConn1 -- F/RConn1
  Axle/LConn2 -- Transform Roller Left/RConn1
  Transform Roller Right/LConn1 -- Axle/LConn1
  Roller Right/RConn1 -- Transform Roller Right/RConn1
  Transform Roller Left/LConn1 -- Roller Left/RConn1

== system sm_trackV_lib_belt_underc_elem/Sprocket No Contact ==
  Roller : Subsystem
  Spokes : Subsystem
  S : PMIOPort  Side=Right
  connections:
  Spokes/LConn21 -- Roller/RConn21
  Spokes/LConn20 -- Roller/RConn20
  Spokes/LConn19 -- Roller/RConn19
  Spokes/LConn18 -- Roller/RConn18
  Spokes/LConn17 -- Roller/RConn17
  Spokes/LConn16 -- Roller/RConn16
  Spokes/LConn15 -- Roller/RConn15
  Spokes/LConn14 -- Roller/RConn14
  Spokes/LConn13 -- Roller/RConn13
  Spokes/LConn12 -- Roller/RConn12
  Spokes/LConn11 -- Roller/RConn11
  Spokes/LConn10 -- Roller/RConn10
  Spokes/LConn9 -- Roller/RConn9
  Spokes/LConn8 -- Roller/RConn8
  Spokes/LConn7 -- Roller/RConn7
  Spokes/LConn6 -- Roller/RConn6
  Spokes/LConn5 -- Roller/RConn5
  Spokes/LConn4 -- Roller/RConn4
  Spokes/LConn3 -- Roller/RConn3
  Spokes/LConn2 -- Roller/RConn2
  Spokes/LConn1 -- Roller/RConn1
  Roller/LConn1 -- S/RConn1

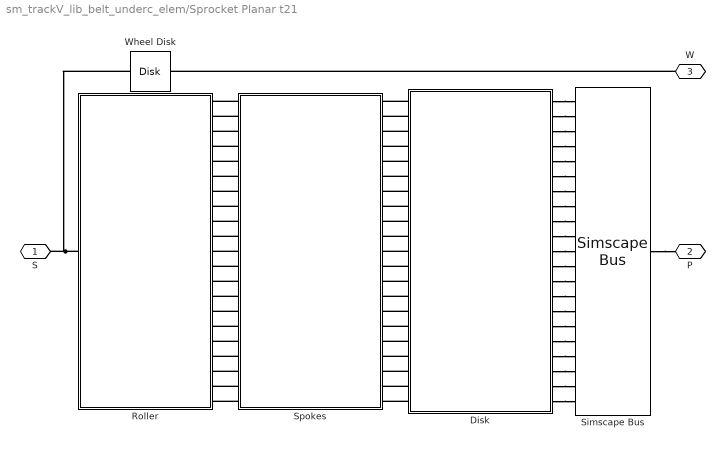
== system sm_trackV_lib_belt_underc_elem/Sprocket Planar t21 ==
  Disk : Subsystem
  Roller : Subsystem
  Simscape Bus : SimscapeBus  HierarchyStrings=P00;P01;P02;P03;P04;P05;P06;P07;P08;P09;P10;P11;P12;P13;P14;P15;P16;P17;P18;P19;P20
  Spokes : Subsystem
  Wheel Disk : sm_lib/Curves and Surfaces/Disk  Radius=sprk_rad_roll  RadiusUnits=m  GraphicType=FromGeometry  GraphicVisPropType=SimpleVisualProperties  GraphicDiffuseColor=sprk_contgeo_roller_clr  GraphicOpacity=sprk_contgeo_roller_opc  GraphicSpecularColor=[0.5 0.5 0.5 1.0]  GraphicAmbientColor=[0.15 0.15 0.15 1.0]  GraphicEmissiveColor=[0.0 0.0 0.0 1.0]  GraphicShininess=75
  S : PMIOPort  Side=Right
  P : PMIOPort  Port=2  Side=Left
  W : PMIOPort  Port=3  Side=Left
  connections:
  Simscape Bus/RConn1 -- P/RConn1
  W/RConn1 -- Wheel Disk/RConn1
  Wheel Disk/LConn1 -- Roller/LConn1 -- S/RConn1
  Spokes/LConn1 -- Roller/RConn1
  Spokes/LConn2 -- Roller/RConn2
  Spokes/LConn3 -- Roller/RConn3
  Spokes/LConn4 -- Roller/RConn4
  Spokes/LConn5 -- Roller/RConn5
  Spokes/LConn6 -- Roller/RConn6
  Spokes/LConn7 -- Roller/RConn7
  Spokes/LConn8 -- Roller/RConn8
  Spokes/LConn9 -- Roller/RConn9
  Spokes/LConn10 -- Roller/RConn10
  Spokes/LConn11 -- Roller/RConn11
  Spokes/LConn12 -- Roller/RConn12
  Spokes/LConn13 -- Roller/RConn13
  Spokes/LConn14 -- Roller/RConn14
  Spokes/LConn15 -- Roller/RConn15
  Spokes/LConn16 -- Roller/RConn16
  Spokes/LConn17 -- Roller/RConn17
  Spokes/LConn18 -- Roller/RConn18
  Spokes/LConn19 -- Roller/RConn19
  Spokes/LConn20 -- Roller/RConn20
  Spokes/LConn21 -- Roller/RConn21
  Disk/LConn1 -- Spokes/RConn1
  Disk/RConn1 -- Simscape Bus/LConn1
  Disk/LConn2 -- Spokes/RConn2
  Disk/RConn2 -- Simscape Bus/LConn2
  Disk/LConn3 -- Spokes/RConn3
  Disk/RConn3 -- Simscape Bus/LConn3
  Disk/LConn4 -- Spokes/RConn4
  Disk/RConn4 -- Simscape Bus/LConn4
  Disk/LConn5 -- Spokes/RConn5
  Disk/RConn5 -- Simscape Bus/LConn5
  Disk/LConn6 -- Spokes/RConn6
  Disk/RConn6 -- Simscape Bus/LConn6
  Disk/LConn7 -- Spokes/RConn7
  Disk/RConn7 -- Simscape Bus/LConn7
  Disk/LConn8 -- Spokes/RConn8
  Disk/RConn8 -- Simscape Bus/LConn8
  Disk/LConn9 -- Spokes/RConn9
  Disk/RConn9 -- Simscape Bus/LConn9
  Disk/LConn10 -- Spokes/RConn10
  Disk/RConn10 -- Simscape Bus/LConn10
  Disk/LConn11 -- Spokes/RConn11
  Disk/RConn11 -- Simscape Bus/LConn11
  Disk/LConn12 -- Spokes/RConn12
  Disk/RConn12 -- Simscape Bus/LConn12
  Disk/LConn13 -- Spokes/RConn13
  Disk/RConn13 -- Simscape Bus/LConn13
  Disk/LConn14 -- Spokes/RConn14
  Disk/RConn14 -- Simscape Bus/LConn14
  Disk/LConn15 -- Spokes/RConn15
  Disk/RConn15 -- Simscape Bus/LConn15
  Disk/LConn16 -- Spokes/RConn16
  Disk/RConn16 -- Simscape Bus/LConn16
  Disk/LConn17 -- Spokes/RConn17
  Disk/RConn17 -- Simscape Bus/LConn17
  Disk/LConn18 -- Spokes/RConn18
  Disk/RConn18 -- Simscape Bus/LConn18
  Disk/LConn19 -- Spokes/RConn19
  Disk/RConn19 -- Simscape Bus/LConn19
  Disk/LConn20 -- Spokes/RConn20
  Disk/RConn20 -- Simscape Bus/LConn20
  Disk/LConn21 -- Spokes/RConn21
  Disk/RConn21 -- Simscape Bus/LConn21

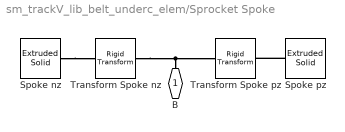
== system sm_trackV_lib_belt_underc_elem/Sprocket Spoke ==
  Spoke nz : sm_lib/Body Elements/Extruded Solid  ExtrusionType=General  PolygonNumSides=3  PolygonOuterRadius=1  PolygonOuterRadiusUnits=m  ExportEntireGeometry=off  ExtrusionCrossSection=spoke_xc  ExtrusionCrossSectionUnits=m  ExportConvexHullGeometry=off  ExtrusionLength=spoke_thk  ExtrusionLengthUnits=m  InertiaType=CalculateFromGeometry  BasedOnType=Density  Density=1000  DensityUnits=kg/m^3  Mass=1  MassUnits=kg  CenterOfMass=[0 0 0]  CenterOfMassUnits=m  MomentsOfInertia=[1 1 1]  MomentsOfInertiaUnits=kg*m^2  ProductsOfInertia=[0 0 0]  ProductsOfInertiaUnits=kg*m^2  GraphicType=FromGeometry  MarkerShape=Sphere  MarkerSize=10  GraphicVisPropType=SimpleVisualProperties  GraphicDiffuseColor=spoke_clr  GraphicOpacity=spoke_opc  GraphicSpecularColor=[0.5 0.5 0.5 1.0]  GraphicAmbientColor=[0.15 0.15 0.15 1.0]  GraphicEmissiveColor=[0.0 0.0 0.0 1.0]  GraphicShininess=75  DoExposeReferenceFrame=on  SerializedFrames=<Frames/>
  Spoke pz : sm_lib/Body Elements/Extruded Solid  ExtrusionType=General  PolygonNumSides=3  PolygonOuterRadius=1  PolygonOuterRadiusUnits=m  ExportEntireGeometry=off  ExtrusionCrossSection=spoke_xc  ExtrusionCrossSectionUnits=m  ExportConvexHullGeometry=off  ExtrusionLength=spoke_thk  ExtrusionLengthUnits=m  InertiaType=CalculateFromGeometry  BasedOnType=Density  Density=1000  DensityUnits=kg/m^3  Mass=1  MassUnits=kg  CenterOfMass=[0 0 0]  CenterOfMassUnits=m  MomentsOfInertia=[1 1 1]  MomentsOfInertiaUnits=kg*m^2  ProductsOfInertia=[0 0 0]  ProductsOfInertiaUnits=kg*m^2  GraphicType=FromGeometry  MarkerShape=Sphere  MarkerSize=10  GraphicVisPropType=SimpleVisualProperties  GraphicDiffuseColor=spoke_clr  GraphicOpacity=spoke_opc  GraphicSpecularColor=[0.5 0.5 0.5 1.0]  GraphicAmbientColor=[0.15 0.15 0.15 1.0]  GraphicEmissiveColor=[0.0 0.0 0.0 1.0]  GraphicShininess=75  DoExposeReferenceFrame=on  SerializedFrames=<Frames/>
  Transform Spoke nz : sm_lib/Frames and Transforms/Rigid Transform  RotationMethod=None  FollAlignAxisA=+X  BaseAlignAxisA=+Y  FollAlignAxisB=+Y  BaseAlignAxisB=+Z  RotationStandardAxis=+Z  RotationAngle=0.0  RotationAngleUnits=deg  RotationArbitraryAxis=[0 0 1]  RotationSequenceAxes=FollowerAxes  RotationSequence=XYX  RotationSequenceAngles=[0 0 0]  RotationSequenceAnglesUnits=deg  RotationMatrix=[1 0 0; 0 1 0; 0 0 1]  Quaternion=[1 0 0 0]  TranslationMethod=StandardAxis  TranslationCartesianOffset=[0 0 0]  TranslationCartesianOffsetUnits=m  TranslationStandardAxis=+Z  TranslationStandardOffset=-spoke_offset  TranslationStandardOffsetUnits=m  TranslationROffset=0  TranslationROffsetUnits=m  TranslationThetaOffset=0  TranslationThetaOffsetUnits=deg  TranslationZOffset=0  TranslationZOffsetUnits=m
  Transform Spoke pz : sm_lib/Frames and Transforms/Rigid Transform  RotationMethod=None  FollAlignAxisA=+X  BaseAlignAxisA=+Y  FollAlignAxisB=+Y  BaseAlignAxisB=+Z  RotationStandardAxis=+Z  RotationAngle=0.0  RotationAngleUnits=deg  RotationArbitraryAxis=[0 0 1]  RotationSequenceAxes=FollowerAxes  RotationSequence=XYX  RotationSequenceAngles=[0 0 0]  RotationSequenceAnglesUnits=deg  RotationMatrix=[1 0 0; 0 1 0; 0 0 1]  Quaternion=[1 0 0 0]  TranslationMethod=StandardAxis  TranslationCartesianOffset=[0 0 0]  TranslationCartesianOffsetUnits=m  TranslationStandardAxis=+Z  TranslationStandardOffset=spoke_offset  TranslationStandardOffsetUnits=m  TranslationROffset=0  TranslationROffsetUnits=m  TranslationThetaOffset=0  TranslationThetaOffsetUnits=deg  TranslationZOffset=0  TranslationZOffsetUnits=m
  B : PMIOPort  Side=Left
  connections:
  Spoke nz/RConn1 -- Transform Spoke nz/RConn1
  Transform Spoke nz/LConn1 -- Transform Spoke pz/LConn1 -- B/RConn1
  Spoke pz/RConn1 -- Transform Spoke pz/RConn1

== system sm_trackV_lib_belt_underc_elem/Tensioner Cyl Roller Frame ==
  Cylinder : sm_lib/Body Elements/Cylindrical Solid  CylinderRadius=cyl_rad  CylinderRadiusUnits=m  CylinderLength=cyl_len  CylinderLengthUnits=m  ExportEntireGeometry=off  InertiaType=CalculateFromGeometry  BasedOnType=Density  Density=cyl_rho  DensityUnits=kg/m^3  Mass=1  MassUnits=kg  CenterOfMass=[0 0 0]  CenterOfMassUnits=m  MomentsOfInertia=[1 1 1]  MomentsOfInertiaUnits=kg*m^2  ProductsOfInertia=[0 0 0]  ProductsOfInertiaUnits=kg*m^2  GraphicType=FromGeometry  MarkerShape=Sphere  MarkerSize=10  GraphicVisPropType=SimpleVisualProperties  GraphicDiffuseColor=cyl_clr  GraphicOpacity=cyl_opc  GraphicSpecularColor=[0.5 0.5 0.5 1.0]  GraphicAmbientColor=[0.15 0.15 0.15 1.0]  GraphicEmissiveColor=[0.0 0.0 0.0 1.0]  GraphicShininess=75  DoExposeReferenceFrame=off  SerializedFrames=<Frames><Frame><Id>Frame2</Id><Value><Name>B</Name><Origin><Source>GeometricFeature</Source><FeatureName>bottom surface</FeatureName></Origin><PrimaryAxis><DefinedDirection>+Z</DefinedDirection><Source>ReferenceFrame</Source><SourceDirection>+Z</SourceDirection><FeatureName></FeatureName></PrimaryAxis><SecondaryAxis><DefinedDirection>+X</DefinedDirection><Source>ReferenceFrame</Source><SourceDirection>+X</SourceDirection><FeatureName></FeatureName></SecondaryAxis></Value></Frame></Frames>
  B : PMIOPort  Side=Left
  F : PMIOPort  Port=2  Side=Right
  connections:
  F/RConn1 -- Cylinder/LConn1 -- B/RConn1

== system sm_trackV_lib_belt_underc_elem/Tensioner Piston Roller Frame ==
  Bracket : Subsystem
  Piston : sm_lib/Body Elements/Cylindrical Solid  CylinderRadius=pist_rad  CylinderRadiusUnits=m  CylinderLength=pist_len  CylinderLengthUnits=m  ExportEntireGeometry=off  InertiaType=CalculateFromGeometry  BasedOnType=Density  Density=pist_rho  DensityUnits=kg/m^3  Mass=1  MassUnits=kg  CenterOfMass=[0 0 0]  CenterOfMassUnits=m  MomentsOfInertia=[1 1 1]  MomentsOfInertiaUnits=kg*m^2  ProductsOfInertia=[0 0 0]  ProductsOfInertiaUnits=kg*m^2  GraphicType=FromGeometry  MarkerShape=Sphere  MarkerSize=10  GraphicVisPropType=SimpleVisualProperties  GraphicDiffuseColor=pist_clr  GraphicOpacity=pist_opc  GraphicSpecularColor=[0.5 0.5 0.5 1.0]  GraphicAmbientColor=[0.15 0.15 0.15 1.0]  GraphicEmissiveColor=[0.0 0.0 0.0 1.0]  GraphicShininess=75  DoExposeReferenceFrame=off  SerializedFrames=<Frames><Frame><Id>Frame2</Id><Value><Name>BracketEnd</Name><Origin><Source>GeometricFeature</Source><FeatureName>top surface</FeatureName></Origin><PrimaryAxis><DefinedDirection>+Z</DefinedDirection><Source>ReferenceFrame</Source><SourceDirection>+Z</SourceDirection><FeatureName></FeatureName></PrimaryAxis><SecondaryAxis><DefinedDirection>+X</DefinedDirection><Source>ReferenceFrame</Source><SourceDirection>+X</SourceDirection><FeatureName></FeatureName></SecondaryAxis></Value></Frame><Frame><Id>Frame3</Id><Value><Name>B</Name><Origin><Source>GeometricFeature</Source><FeatureName>bottom surface</FeatureName></Origin><PrimaryAxis><DefinedDirection>+Z</DefinedDirection><Source>ReferenceFrame</Source><SourceDirection>+Z</SourceDirection><FeatureName></FeatureName></PrimaryAxis><SecondaryAxis><DefinedDirection>+X</DefinedDirection><Source>ReferenceFrame</Source><SourceDirection>+X</SourceDirection><FeatureName></FeatureName></SecondaryAxis></Value></Frame></Frames>
  "Transform Revolute to Prismatic " : sm_lib/Frames and Transforms/Rigid Transform  RotationMethod=AlignedAxes  FollAlignAxisA=+Z  BaseAlignAxisA=+Y  FollAlignAxisB=+Y  BaseAlignAxisB=+X  RotationStandardAxis=+Z  RotationAngle=0.0  RotationAngleUnits=deg  RotationArbitraryAxis=[0 0 1]  RotationSequenceAxes=FollowerAxes  RotationSequence=XYX  RotationSequenceAngles=[0 0 0]  RotationSequenceAnglesUnits=deg  RotationMatrix=[1 0 0; 0 1 0; 0 0 1]  Quaternion=[1 0 0 0]  TranslationMethod=None  TranslationCartesianOffset=[0 0 0]  TranslationCartesianOffsetUnits=m  TranslationStandardAxis=+Z  TranslationStandardOffset=0.4  TranslationStandardOffsetUnits=m  TranslationROffset=0  TranslationROffsetUnits=m  TranslationThetaOffset=0  TranslationThetaOffsetUnits=deg  TranslationZOffset=0  TranslationZOffsetUnits=m
  a : PMIOPort  Side=Right
  Cyl : PMIOPort  Port=2  Side=Left
  connections:
  "Transform Revolute to Prismatic "/LConn1 -- Bracket/RConn1
  Piston/LConn1 -- Bracket/LConn1
  Cyl/RConn1 -- Piston/RConn1
  "Transform Revolute to Prismatic "/RConn1 -- a/RConn1
